simulink model "VSD_Motor_20kW"  (Simulink 9.3)
settings: Solver=ode23t  StartTime=0.0  StopTime=2  FixedStep=1e-5  MaxStep=1e-5  MinStep=1e-7  RelTol=1e-6  AbsTol=1e-6  EnableMultiTasking=on
libraries: powerlib x24, powerlib_extras x6, simulink x2
(part 2 of 2)

== system VSD_Motor_20kW/Rectifier AC-DC/Control scheme/SVPWM/time convert2 ==
  Ta : Inport
  Tb : Inport  Port=2
  Tc : Inport  Port=3
  N : Inport  Port=4
  Multiport Switch1 : MultiPortSwitch  Inputs=6
  Multiport Switch2 : MultiPortSwitch  Inputs=6
  Multiport Switch3 : MultiPortSwitch  Inputs=6
  Tcm1 : Outport
  Tcm2 : Outport  Port=2
  Tcm3 : Outport  Port=3
  wires:
  Tb/1 -> Multiport Switch2/7, Multiport Switch2/2, Multiport Switch3/6, Multiport Switch3/3, Multiport Switch1/5, Multiport Switch1/4
  Ta/1 -> Multiport Switch3/7, Multiport Switch3/5, Multiport Switch1/6, Multiport Switch1/2, Multiport Switch2/4, Multiport Switch2/3
  Tc/1 -> Multiport Switch2/6, Multiport Switch2/5, Multiport Switch1/7, Multiport Switch3/4, Multiport Switch3/2, Multiport Switch1/3
  Multiport Switch2/1 -> Tcm1/1
  Multiport Switch1/1 -> Tcm2/1
  Multiport Switch3/1 -> Tcm3/1
  N/1 -> Multiport Switch3/1, Multiport Switch2/1, Multiport Switch1/1
